simulink model "sampleModel2007_3"  (R2023a)
settings: Solver=VariableStepAuto  StartTime=0.0  StopTime=10.0  RelTol=1e-3
libraries: simulink x4, hdlsllib x2
settings Model: Creator=user1  LastModifiedBy=user1

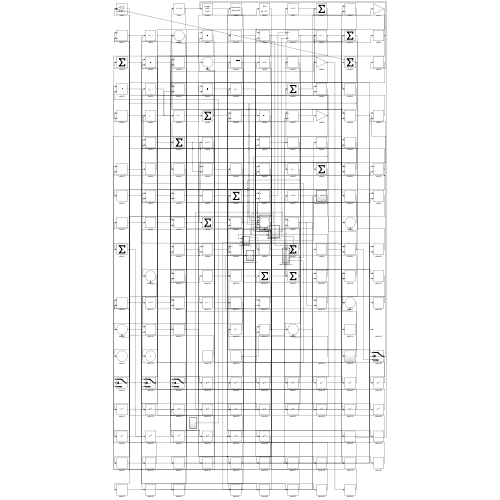
[thumbnail: Simulink's stored preview of the top-level diagram]
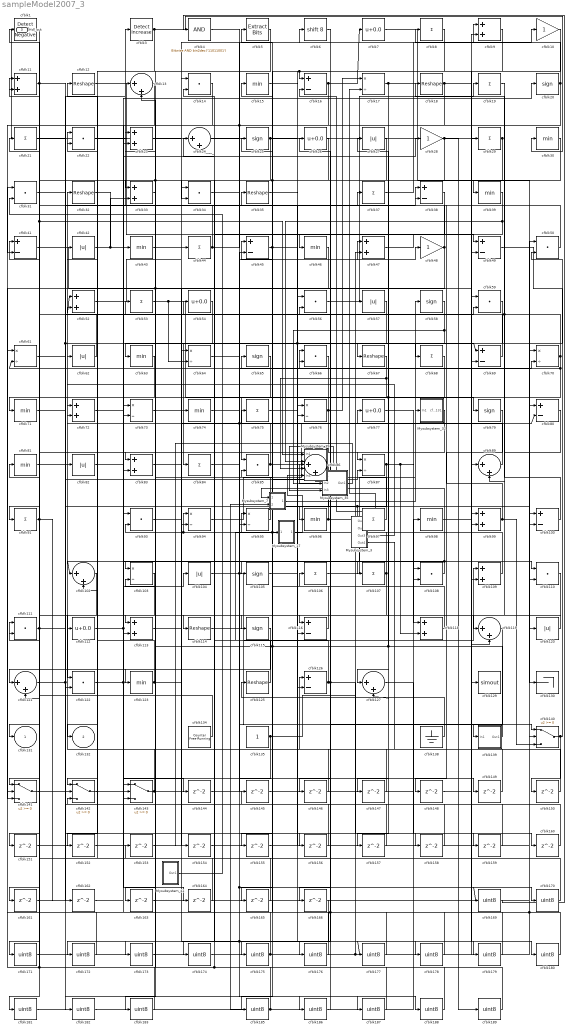
== system sampleModel2007_3 ==
  Mysubsystem_17 : Subsystem  TreatAsAtomicUnit=on  RTWFcnName=Mysubsystem_17
      settings: RTWFcnNameOpts=User specified  RTWFileNameOpts=Use function name
  Mysubsystem_3 : Subsystem  TreatAsAtomicUnit=on  RTWFcnName=Mysubsystem_3
      settings: RTWFcnNameOpts=User specified  RTWFileNameOpts=Use function name
  Mysubsystem_32 : Subsystem  TreatAsAtomicUnit=on  RTWFcnName=Mysubsystem_32
      settings: RTWFcnNameOpts=User specified  RTWFileNameOpts=Use function name
  Mysubsystem_35 : Subsystem  TreatAsAtomicUnit=on  RTWFcnName=Mysubsystem_35
      settings: RTWFcnNameOpts=User specified  RTWFileNameOpts=Use function name
  Mysubsystem_39 : Subsystem  TreatAsAtomicUnit=on  RTWFcnName=Mysubsystem_39
      settings: RTWFcnNameOpts=User specified  RTWFileNameOpts=Use function name
  Mysubsystem_41 : Subsystem  TreatAsAtomicUnit=on  RTWFcnName=Mysubsystem_41
      settings: RTWFcnNameOpts=User specified  RTWFileNameOpts=Use function name
  Mysubsystem_7 : Subsystem  TreatAsAtomicUnit=on  RTWFcnName=Mysubsystem_7
      settings: RTWFcnNameOpts=User specified  RTWFileNameOpts=Use function name
  cfblk1 : hdlsllib/Logic and Bit Operations/Detect Fall Negative  vinit=0  OutDataTypeStr=uint8
  cfblk10 : Gain  OutDataTypeStr=uint8
  cfblk{16,38,41,45,49,69,80,100,116,126} (10 alike) : Sum  Inputs=+-  OutDataTypeStr=uint8
  cfblk{13,24,86,89,102,119,121,127} (8 alike) : Sum  Inputs=|++  OutDataTypeStr=uint8
  cfblk{17,61,64,70,73,76,87,94..95,103} (10 alike) : Product  Inputs=*/  OutDataTypeStr=uint8  RndMeth=Zero  SaturateOnIntegerOverflow=on
  cfblk{27,42,57,62,82,104,120} (7 alike) : Abs  OutDataTypeStr=uint8  SaturateOnIntegerOverflow=off
  cfblk{20,25,58,65,79,105,115} (7 alike) : Signum
  cfblk{8,19,21,29,37,44,53,68,75,84,91,97,106..107} (14 alike) : Sum  Inputs=+  OutDataTypeStr=uint8
  cfblk{14,22,31,34,50,56,59,66,85,93,108,110..111,122} (14 alike) : DotProduct  OutDataTypeStr=uint8
  cfblk{9,11,23,33,47,52,72,83,99,109,113,118} (12 alike) : Sum  OutDataTypeStr=uint8
  cfblk{7,26,54,77,112} (5 alike) : Bias  Bias=0.0  SaturateOnIntegerOverflow=off
  cfblk{12,18,32,35,67,114,125} (7 alike) : Reshape
  cfblk{15,30,39,43,46,63,71,74,81,96,98,123} (12 alike) : MinMax  OutDataTypeStr=uint8
  cfblk129 : ToWorkspace  VariableName=simout  SaveFormat=Timeseries  SampleTime=-1
  cfblk130 : Terminator
  cfblk134 : hdlsllib/Sources/Counter Free-Running  NumBits=16  tsamp=-1
  cfblk135 : Constant  OutDataTypeStr=uint8  SampleTime=-1
  cfblk138 : Ground
  cfblk139 : Subsystem
      settings: LibrarySourceBlock=|
      | hdlsllib/Ports &
      | Subsystems/Subsystem
  cfblk{140..143} (4 alike) : Switch  OutDataTypeStr=uint8  SaturateOnIntegerOverflow=off  InputSameDT=off
  cfblk{144..166} (23 alike) : Delay  SampleTime=1
  cfblk{169..183,185..189} (20 alike) : DataTypeConversion  OutDataTypeStr=uint8  SaturateOnIntegerOverflow=off  RndMeth=Floor
  cfblk28 : Gain  OutDataTypeStr=uint8
  cfblk3 : simulink/Logic and Bit Operations/Detect Increase  vinit=0.0  OutDataTypeStr=uint8
      settings: LibrarySourceBlock=|
      | hdlsllib/Logic and Bit
      | Operations/Detect
      | Increase
  cfblk4 : simulink/Logic and Bit Operations/Bitwise Operator  logicop=AND  UseBitMask=on  BitMask=bin2dec('11011001')  BitMaskRealWorld=Stored Integer
      settings: LibrarySourceBlock=|
      | hdlsllib/Logic and Bit
      | Operations/Bitwise
      | Operator
  cfblk48 : Gain  OutDataTypeStr=uint8
  cfblk5 : simulink/Logic and Bit Operations/Extract Bits  bitsToExtract=Upper half  numBits=8  bitIdxRange=[0 7]  outScalingMode=Preserve fixed-point scaling
      settings: LibrarySourceBlock=|
      | hdlsllib/Logic and Bit
      | Operations/Extract Bits
  cfblk6 : ArithShift  BitShiftNumber=8
  cfblk131 : Outport  OutDataTypeStr=uint8  VectorParamsAs1DForOutWhenUnconnected=off
  cfblk132 : Outport  Port=2  OutDataTypeStr=uint8  VectorParamsAs1DForOutWhenUnconnected=off
  Hdl_out : Outport  Port=3  OutDataTypeStr=uint8
  wires:
  cfblk97/1 -> cfblk65/1
  cfblk49/1 -> cfblk84/1
  cfblk87/1 -> cfblk97/1, cfblk155/1, cfblk110/1, cfblk118/2
  cfblk68/1 -> cfblk85/1
  cfblk32/1 -> cfblk43/1
  cfblk143/1 -> cfblk32/1, cfblk45/2
  cfblk83/1 -> cfblk77/1
  cfblk17/1 -> cfblk87/1, cfblk130/1
  cfblk7/1 -> cfblk39/1
  cfblk140/1 -> cfblk50/2, cfblk150/1
  cfblk76/1 -> cfblk71/1, cfblk17/1, cfblk121/2
  cfblk12/1 -> cfblk46/1
  cfblk107/1 -> cfblk13/2, cfblk94/1, cfblk5/1, cfblk163/1
  cfblk134/1 -> cfblk111/1
  cfblk5/1 -> cfblk63/1
  cfblk118/1 -> cfblk35/1
  cfblk114/1 -> cfblk109/1
  cfblk18/1 -> cfblk129/1, cfblk41/2
  cfblk116/1 -> cfblk106/1
  cfblk16/1 -> cfblk7/1, cfblk33/1
  cfblk106/1 -> cfblk58/1
  cfblk8/1 -> cfblk16/1, cfblk165/1
  cfblk102/1 -> cfblk122/1
  cfblk42/1 -> cfblk107/1, cfblk33/2
  cfblk14/1 -> cfblk142/1
  cfblk50/1 -> cfblk3/1
  cfblk45/1 -> cfblk69/2, cfblk99/2, cfblk25/1
  cfblk86/1 -> cfblk185/1
  cfblk91/1 -> cfblk121/1, cfblk162/1
  cfblk27/1 -> Mysubsystem_39/1(In1), cfblk161/1, cfblk105/1
  cfblk81/1 -> cfblk188/1
  cfblk46/1 -> cfblk141/3, cfblk183/1
  cfblk105/1 -> cfblk48/1
  cfblk20/1 -> cfblk132/1, cfblk95/2, cfblk8/1
  cfblk53/1 -> cfblk79/1, cfblk64/2
  cfblk52/1 -> cfblk14/1
  cfblk59/1 -> cfblk67/1
  cfblk33/1 -> cfblk83/1
  cfblk125/1 -> cfblk14/2
  cfblk22/1 -> cfblk99/1
  cfblk126/1 -> Mysubsystem_17/1(In1), cfblk66/1, cfblk160/1
  cfblk66/1 -> cfblk83/2
  cfblk84/1 -> cfblk70/2
  cfblk108/1 -> Mysubsystem_7/1(In1), cfblk102/1
  cfblk63/1 -> cfblk112/1
  cfblk3/1 -> cfblk30/1, cfblk152/1
  cfblk123/1 -> cfblk22/1, cfblk156/1
  cfblk11/1 -> cfblk96/1, cfblk69/1, cfblk91/1
  cfblk93/1 -> cfblk175/1
  cfblk141/1 -> cfblk13/1
  cfblk98/1 -> cfblk180/1
  cfblk44/1 -> cfblk12/1, cfblk6/1
  cfblk23/1 -> cfblk9/1
  cfblk48/1 -> cfblk11/1, cfblk94/2
  cfblk89/1 -> cfblk53/1
  cfblk80/1 -> cfblk119/1
  cfblk70/1 -> cfblk127/2, cfblk181/1, cfblk61/2, cfblk22/2
  cfblk73/1 -> cfblk74/1
  cfblk100/1 -> cfblk52/1, cfblk18/1
  cfblk28/1 -> cfblk127/1, cfblk189/1
  cfblk121/1 -> cfblk87/2, cfblk158/1
  cfblk85/1 -> cfblk72/1, cfblk50/1
  cfblk82/1 -> cfblk20/1
  cfblk74/1 -> cfblk80/2, cfblk149/1
  cfblk56/1 -> cfblk19/1
  cfblk34/1 -> cfblk177/1, cfblk187/1, cfblk169/1
  cfblk47/1 -> cfblk49/1
  cfblk1/1 -> cfblk171/1
  cfblk111/1 -> cfblk21/1, cfblk186/1
  cfblk41/1 -> cfblk119/2
  cfblk13/1 -> cfblk73/2
  cfblk104/1 -> cfblk139/1(In1), cfblk47/1
  cfblk138/1 -> cfblk125/1
  cfblk43/1 -> cfblk44/1
  cfblk75/1 -> cfblk37/1
  cfblk65/1 -> cfblk123/1
  cfblk67/1 -> Mysubsystem_39/3(In3), cfblk113/1
  cfblk57/1 -> cfblk116/1
  cfblk62/1 -> cfblk41/1
  cfblk71/1 -> cfblk59/2
  cfblk109/1 -> cfblk75/1
  cfblk58/1 -> Mysubsystem_35/2(In2), cfblk68/1
  cfblk61/1 -> cfblk38/1
  cfblk122/1 -> cfblk104/1, cfblk144/1
  cfblk64/1 -> cfblk76/2
  cfblk96/1 -> cfblk118/1, cfblk45/1
  cfblk120/1 -> cfblk115/1
  cfblk39/1 -> Mysubsystem_39/2(In2), cfblk114/1
  cfblk142/1 -> cfblk143/2
  cfblk94/1 -> cfblk9/2
  cfblk10/1 -> cfblk49/2
  cfblk19/1 -> cfblk89/2
  cfblk24/1 -> cfblk140/1
  cfblk99/1 -> cfblk38/2, cfblk140/3
  cfblk77/1 -> cfblk109/2
  cfblk103/1 -> cfblk141/1
  cfblk9/1 -> cfblk126/2
  cfblk139/1(Out1) -> cfblk95/1, cfblk103/2, cfblk27/1
  cfblk25/1 -> cfblk103/1, cfblk113/2, cfblk110/2
  cfblk135/1 -> cfblk143/3, cfblk47/2
  cfblk26/1 -> cfblk34/2
  cfblk95/1 -> cfblk23/1
  cfblk21/1 -> cfblk82/1
  cfblk112/1 -> cfblk28/1, cfblk164/1
  cfblk72/1 -> cfblk100/2
  cfblk37/1 -> cfblk10/1
  cfblk69/1 -> cfblk42/1
  cfblk144/1 -> cfblk116/2
  cfblk145/1 -> cfblk108/1
  cfblk29/1 -> cfblk146/1, Hdl_out/1
  cfblk146/1 -> cfblk102/2
  cfblk38/1 -> cfblk147/1
  cfblk147/1 -> cfblk85/2
  cfblk79/1 -> cfblk148/1
  cfblk148/1 -> cfblk89/1
  cfblk149/1 -> cfblk66/2
  cfblk150/1 -> cfblk24/1
  cfblk115/1 -> cfblk151/1
  cfblk151/1 -> cfblk34/1
  cfblk152/1 -> cfblk23/2
  cfblk153/1 -> cfblk56/1
  cfblk154/1 -> cfblk59/1
  cfblk155/1 -> cfblk70/1
  cfblk156/1 -> cfblk64/1
  cfblk110/1 -> cfblk157/1
  cfblk157/1 -> cfblk76/1
  cfblk158/1 -> cfblk52/2
  cfblk127/1 -> cfblk159/1
  cfblk159/1 -> cfblk142/2
  cfblk160/1 -> cfblk72/2
  cfblk161/1 -> cfblk122/2
  cfblk162/1 -> cfblk143/1
  cfblk163/1 -> cfblk100/1
  cfblk164/1 -> cfblk11/2
  cfblk165/1 -> cfblk142/3
  cfblk6/1 -> cfblk166/1
  cfblk169/1 -> cfblk4/1
  cfblk4/1 -> cfblk170/1
  cfblk170/1 -> cfblk73/1
  cfblk171/1 -> cfblk140/2, cfblk57/1
  cfblk166/1 -> cfblk172/1
  cfblk172/1 -> cfblk1/1
  cfblk54/1 -> cfblk173/1
  cfblk173/1 -> cfblk120/1
  cfblk30/1 -> cfblk174/1
  cfblk174/1 -> cfblk54/1
  cfblk175/1 -> cfblk61/1, cfblk29/1
  cfblk119/1 -> cfblk176/1
  cfblk176/1 -> cfblk93/1
  cfblk177/1 -> cfblk93/2
  cfblk15/1 -> cfblk178/1
  cfblk178/1 -> cfblk26/1
  cfblk113/1 -> cfblk179/1
  cfblk179/1 -> cfblk15/1
  cfblk180/1 -> cfblk145/1, cfblk56/2, cfblk80/1
  cfblk181/1 -> cfblk98/1
  cfblk31/1 -> cfblk182/1
  cfblk182/1 -> cfblk108/2
  cfblk183/1 -> cfblk31/1
  cfblk185/1 -> Mysubsystem_7/2(In2), cfblk153/1, cfblk24/2
  cfblk186/1 -> cfblk86/1
  cfblk187/1 -> cfblk86/2
  cfblk188/1 -> cfblk141/2, cfblk111/2
  cfblk189/1 -> cfblk81/1
  Mysubsystem_3/1(Out1) -> cfblk16/2
  Mysubsystem_3/2(Out2) -> cfblk17/2
  Mysubsystem_3/3(Out3) -> cfblk62/1
  Mysubsystem_3/4(Out4) -> cfblk126/1
  Mysubsystem_7/1(Out1) -> Mysubsystem_32/1(In1)
  Mysubsystem_32/1(cfblk131) -> cfblk131/1
  cfblk35/1 -> Mysubsystem_35/1(In1)
  Mysubsystem_35/1(Out1) -> cfblk154/1
  Mysubsystem_17/1(Out1) -> Mysubsystem_39/4(In4)
  Mysubsystem_39/1(Out1) -> Mysubsystem_35/3(In3)
  Mysubsystem_41/1(Out1) -> cfblk31/2

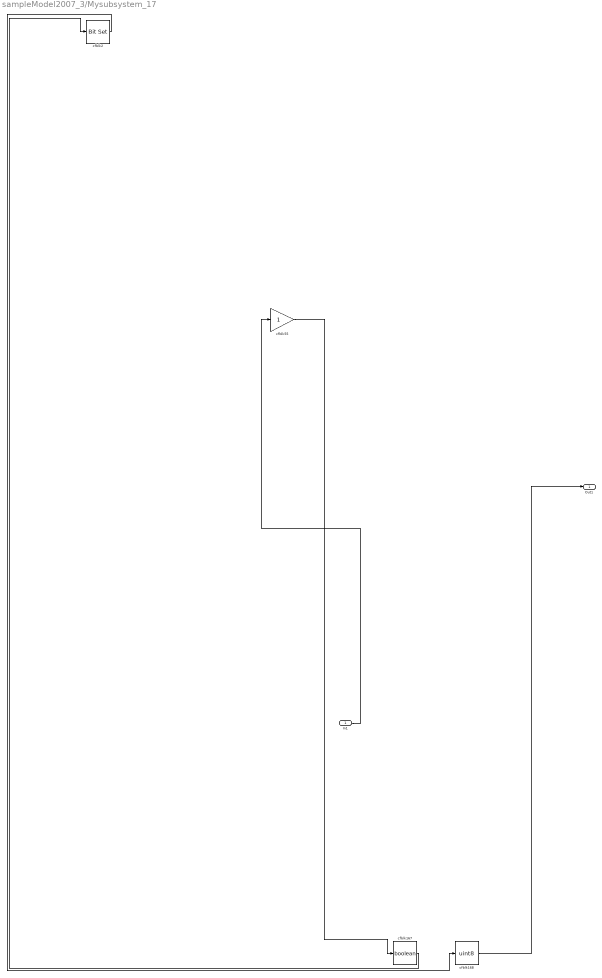
== system sampleModel2007_3/Mysubsystem_17 ==
  In1 : Inport
  cfblk167 : DataTypeConversion  OutDataTypeStr=boolean  SaturateOnIntegerOverflow=off  RndMeth=Floor
  cfblk168 : DataTypeConversion  OutDataTypeStr=uint8  SaturateOnIntegerOverflow=off  RndMeth=Floor
  cfblk2 : simulink/Logic and Bit Operations/Bit Set  iBit=0
      settings: LibrarySourceBlock=|
      | hdlsllib/Logic and Bit
      | Operations/Bit Set
  cfblk55 : Gain
  Out1 : Outport
  wires:
  cfblk55/1 -> cfblk167/1
  cfblk2/1 -> cfblk168/1
  In1/1 -> cfblk55/1
  cfblk167/1 -> cfblk2/1
  cfblk168/1 -> Out1/1

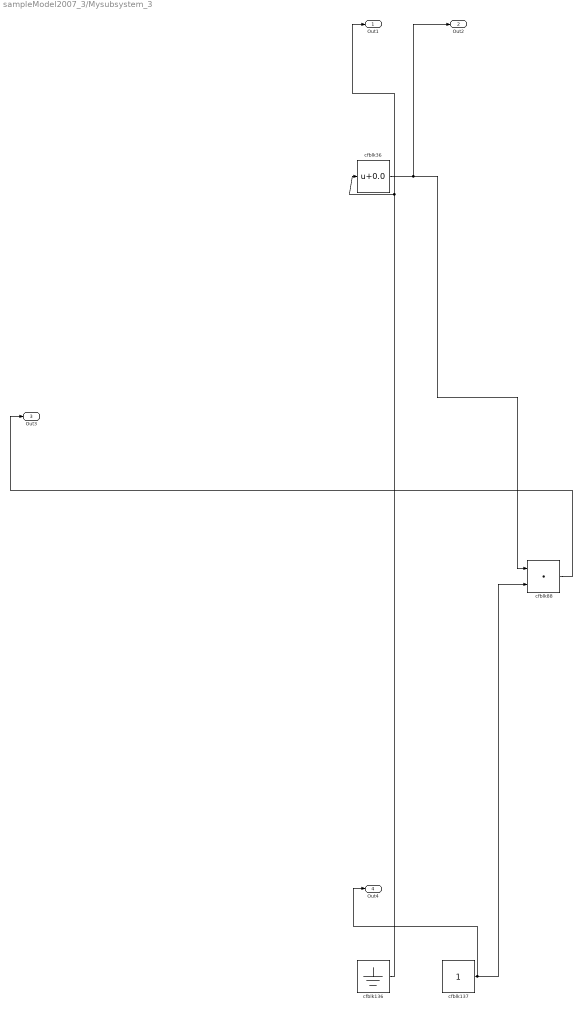
== system sampleModel2007_3/Mysubsystem_3 ==
  cfblk136 : Ground
  cfblk137 : Constant  SampleTime=-1
  cfblk36 : Bias  Bias=0.0  SaturateOnIntegerOverflow=off
  cfblk88 : DotProduct  OutDataTypeStr=Inherit: Inherit via internal rule
  Out1 : Outport
  Out2 : Outport  Port=2
  Out3 : Outport  Port=3
  Out4 : Outport  Port=4
  wires:
  cfblk36/1 -> Out2/1, cfblk88/1
  cfblk88/1 -> Out3/1
  cfblk136/1 -> Out1/1, cfblk36/1
  cfblk137/1 -> Out4/1, cfblk88/2

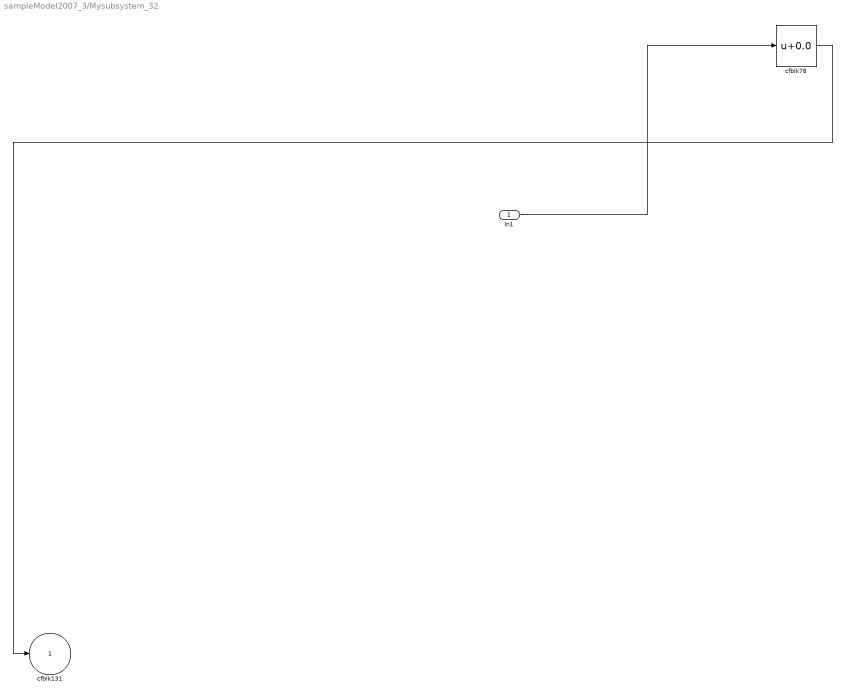
== system sampleModel2007_3/Mysubsystem_32 ==
  In1 : Inport
  cfblk78 : Bias  Bias=0.0  SaturateOnIntegerOverflow=off
  cfblk131 : Outport  VectorParamsAs1DForOutWhenUnconnected=off
  wires:
  cfblk78/1 -> cfblk131/1
  In1/1 -> cfblk78/1

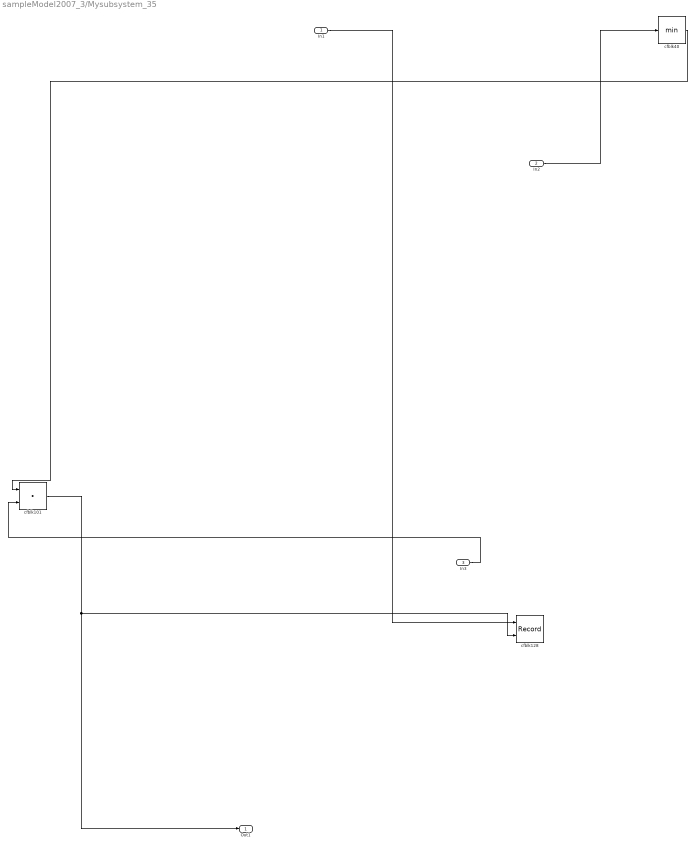
== system sampleModel2007_3/Mysubsystem_35 ==
  In1 : Inport
  In2 : Inport  Port=2
  In3 : Inport  Port=3
  cfblk101 : DotProduct  OutDataTypeStr=Inherit: Inherit via internal rule
  cfblk128 : Record  FileSettingsInternal="{\"entries\":[{\"content\":{\"excelSettings\":{\"content\":{},\"type\":\"Streamout.ExcelSettings\"}},\"type\":\"Streamout.FileSettingStorage\",\"uuid\":\"\"}],\"packageUris\":[\"http:\\/\\/schema.mathworks.com\\/mf0\\/streamout_blocks\\/R2020a\"],\"version\":\"1.0\"}"  Layout=[1 1]  SignalsInternal="{\"entries\":[{\"content\":{},\"type\":\"RecordBlkView.InputSignals\",\"uuid\":\"\"}],\"packageUris\":[\"http:\\/\\/schema.mathworks.com\\/mf0\\/streamout_blocks\\/R2020a\"],\"version\":\"1.0\"}"  VisualizationBindings="{\"xyplotplugin\":{\"info\":[{\"series\":[],\"subplotID\":1}]}}"  CompatibilityTag=XY  st=-1
  cfblk40 : MinMax
  Out1 : Outport
  wires:
  In2/1 -> cfblk40/1
  In3/1 -> cfblk101/2
  cfblk101/1 -> Out1/1, cfblk128/2
  cfblk40/1 -> cfblk101/1
  In1/1 -> cfblk128/1

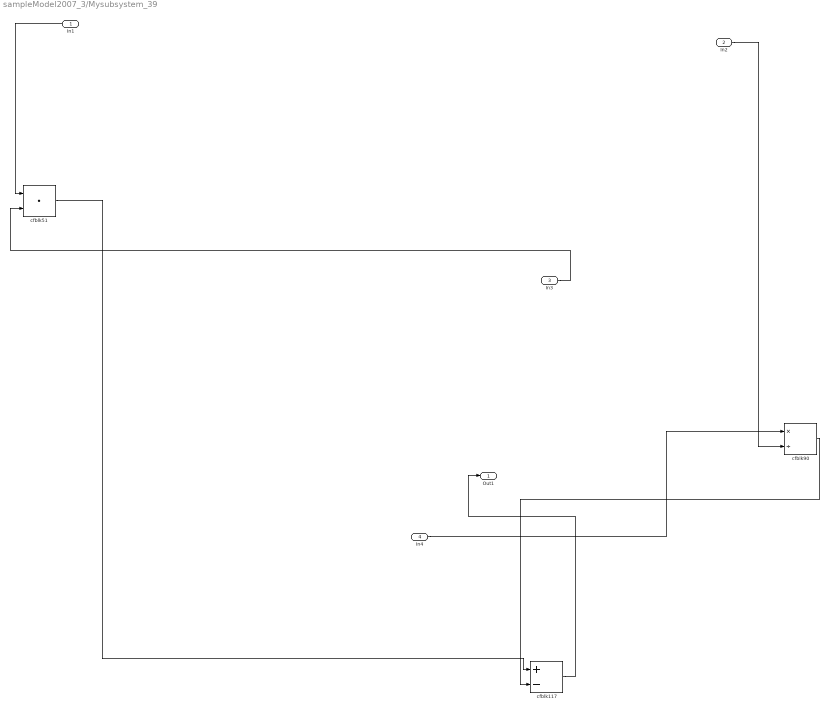
== system sampleModel2007_3/Mysubsystem_39 ==
  In1 : Inport
  In2 : Inport  Port=2
  In3 : Inport  Port=3
  In4 : Inport  Port=4
  cfblk117 : Sum  Inputs=+-
  cfblk51 : DotProduct  OutDataTypeStr=Inherit: Inherit via internal rule
  cfblk90 : Product  Inputs=*/  RndMeth=Zero  SaturateOnIntegerOverflow=on
  Out1 : Outport
  wires:
  In1/1 -> cfblk51/1
  cfblk51/1 -> cfblk117/1
  cfblk117/1 -> Out1/1
  In4/1 -> cfblk90/1
  cfblk90/1 -> cfblk117/2
  In3/1 -> cfblk51/2
  In2/1 -> cfblk90/2

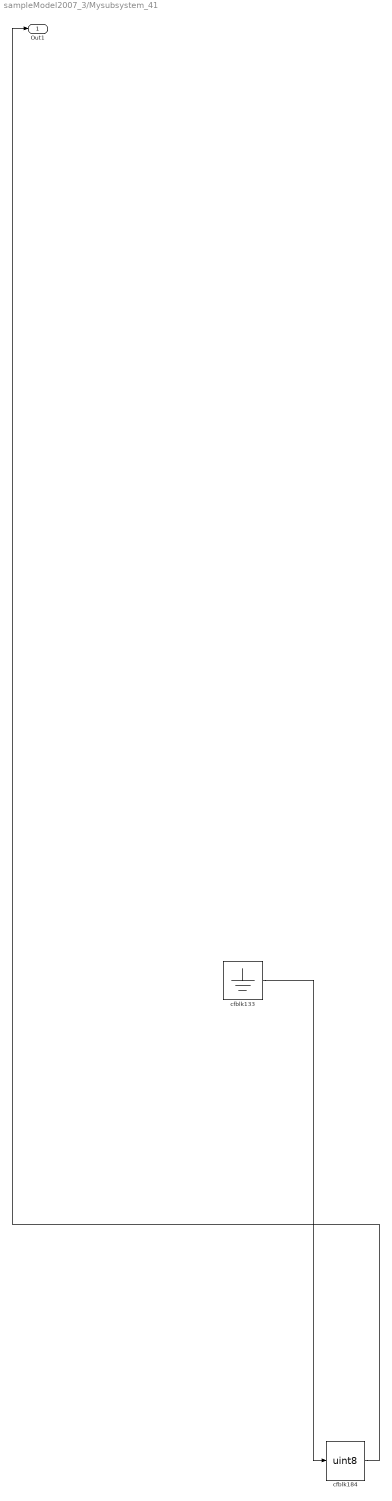
== system sampleModel2007_3/Mysubsystem_41 ==
  cfblk133 : Ground
  cfblk184 : DataTypeConversion  OutDataTypeStr=uint8  SaturateOnIntegerOverflow=off  RndMeth=Floor
  Out1 : Outport
  wires:
  cfblk133/1 -> cfblk184/1
  cfblk184/1 -> Out1/1

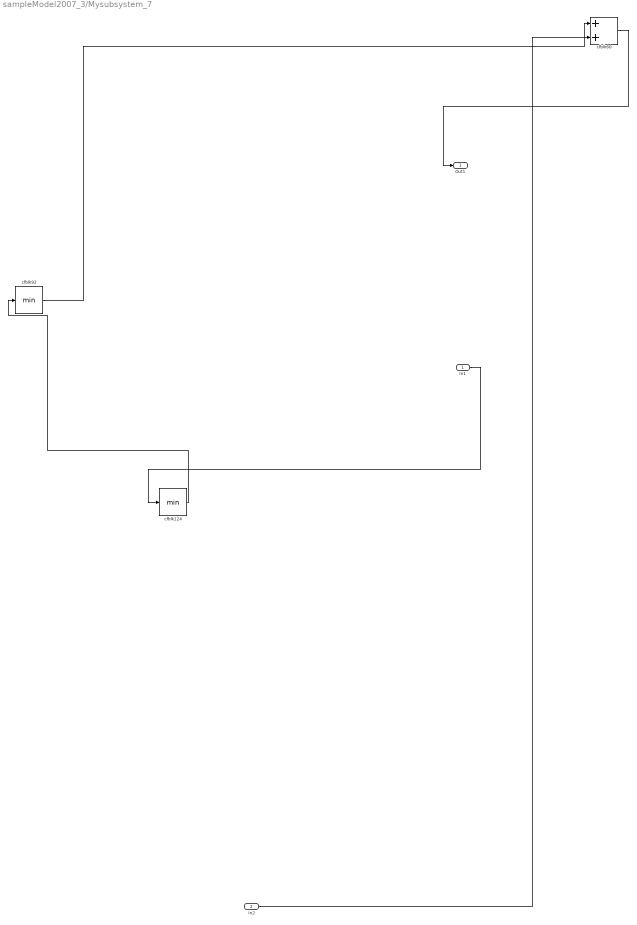
== system sampleModel2007_3/Mysubsystem_7 ==
  In1 : Inport
  In2 : Inport  Port=2
  cfblk124 : MinMax
  cfblk60 : Sum
  cfblk92 : MinMax
  Out1 : Outport
  wires:
  In2/1 -> cfblk60/2
  cfblk92/1 -> cfblk60/1
  cfblk124/1 -> cfblk92/1
  In1/1 -> cfblk124/1
  cfblk60/1 -> Out1/1

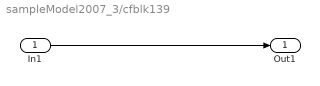
== system sampleModel2007_3/cfblk139 ==
  In1 : Inport
  Out1 : Outport
  wires:
  In1/1 -> Out1/1
